simulink model "Dynamics_Simulation"  (R2023a)
settings: Solver=VariableStepAuto  StartTime=0.0  StopTime=10.0  RelTol=1e-3
libraries: dspinverses x1, DaVinci_LibDynamical x1
settings Model: Creator=afons  LastModifiedBy=afons

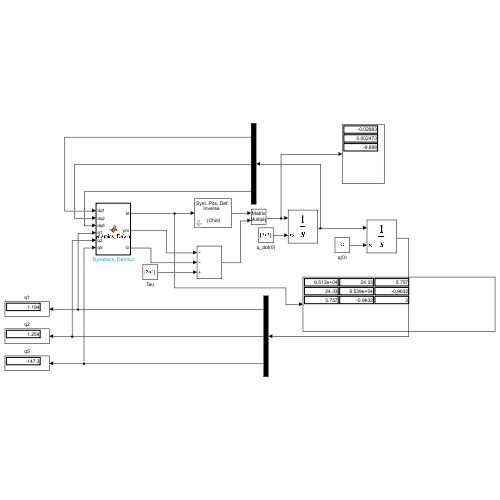
[thumbnail: Simulink's stored preview of the top-level diagram]
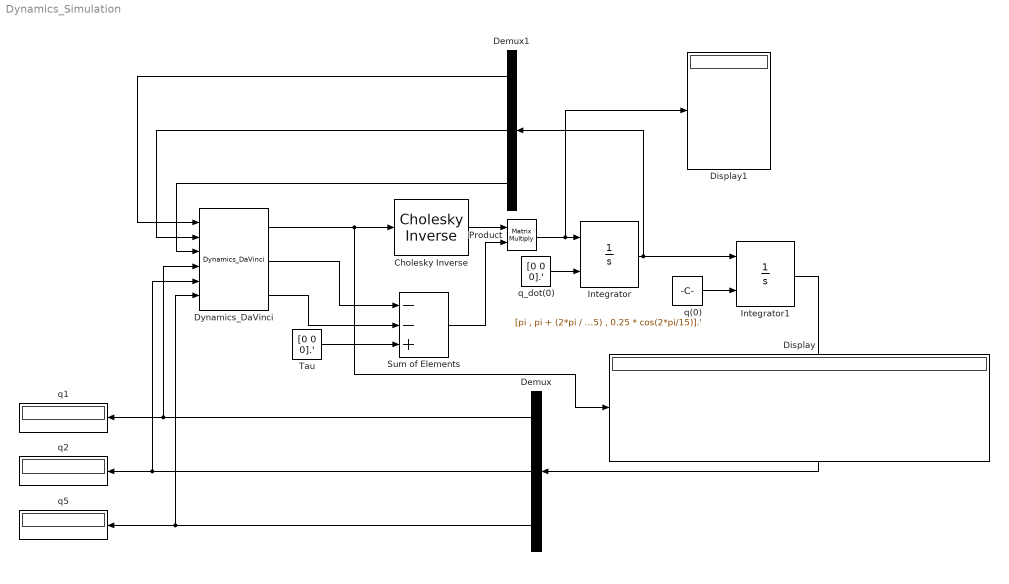
== system Dynamics_Simulation ==
  Cholesky Inverse : dspinverses/Cholesky Inverse  errmode=Warning
  Demux : Demux  Outputs=3
  Demux1 : Demux  Outputs=3
  Display : Display
  Display1 : Display
  Dynamics_DaVinci : DaVinci_LibDynamical/Dynamics_DaVinci  SystemSampleTime=-1  VariantActivationTime=update diagram  Latency=0  AutoFrameSizeCalculation=off
      settings: LibrarySourceBlock=|
      | simulink/User-Defined
      | Functions/MATLAB Function
  Integrator : Integrator  InitialConditionSource=external
  Integrator1 : Integrator  InitialConditionSource=external
  Product : Product  Multiplication=Matrix(*)
  Sum of Elements : Sum  Inputs=--+
  Tau : Constant  Value=[0 0 0].'
  q(0) : Constant  Value=[pi , pi + (2*pi / 15) , 0.25 * cos(2*pi/15)].'
  q1 : Display
  q2 : Display
  q5 : Display
  q_dot(0) : Constant  Value=[0 0 0].'
  wires:
  Integrator/1 -> Demux1/1, Integrator1/1
  Integrator1/1 -> Demux/1
  Sum of Elements/1 -> Product/2
  Product/1 -> Display1/1, Integrator/1
  Tau/1 -> Sum of Elements/3
  q_dot(0)/1 -> Integrator/2
  q(0)/1 -> Integrator1/2
  Dynamics_DaVinci/2 -> Sum of Elements/1
  Dynamics_DaVinci/3 -> Sum of Elements/2
  Demux/3 -> Dynamics_DaVinci/6, q5/1
  Demux/2 -> Dynamics_DaVinci/5, q2/1
  Demux/1 -> Dynamics_DaVinci/4, q1/1
  Demux1/1 -> Dynamics_DaVinci/1
  Demux1/2 -> Dynamics_DaVinci/2
  Demux1/3 -> Dynamics_DaVinci/3
  Dynamics_DaVinci/1 -> Cholesky Inverse/1, Display/1
  Cholesky Inverse/1 -> Product/1
